simulink model "ffb_Cularis_server"  (Simulink 8.6)
settings: Solver=FixedStepAuto  SolverMode=SingleTasking  StartTime=0.0  StopTime=uavsim.simConfig.tsim  FixedStep=uavsim.simConfig.tsample_model  RelTol=1
model workspace (MAT data in the model file):
  VortexSig = Simulink.Signal
  VortexSig.DataType = 'Bus: VortexStates'
  VortexSig.Units = 'auto'
  VortexSig.Dimensions = [10 1]
  VortexSig.DimensionsMode = 'Fixed'
  VortexSig.Complexity = 'real'
  VortexSig.SampleTime = -1
  VortexSig.SamplingMode = 'auto'
  VortexSig.InitialValue = 'VortexStates_MATLABStruct_array'
undefined symbols (not defined in the file or in its folder): uavsim
libraries: uavsimblockset x4, aerolibtransform2 x4, uavsimBlockset_UAV3DInterface x2, aerolibanimutils x1
settings Model: Creator=mstolle  LastModifiedBy=j.bolting  ExtModeTrigDuration=100
settings SolverCC: ZcThreshold=1e-5  ZeroCrossAlgorithm=Adaptive  AlgebraicLoopSolver=LineSearch  AutoInsertRateTranBlk=on
settings DataIOCC: LimitDataPoints=off  SaveFinalState=on  SaveFormat=StructureWithTime  SignalLoggingSaveFormat=Dataset  SaveOutput=off  SaveState=on  DSMLogging=off  InspectSignalLogs=on  StateSaveName=tmp_raccel_xout
settings OptimizationCC: BlockReduction=off  OptimizeBlockIOStorage=off  BufferReuse=off  GlobalBufferReuse=off  ExpressionFolding=off  LocalBlockOutputs=off  EfficientMapNaN2IntZero=off  SimCompilerOptimization=on
settings DebuggingCC: UnderspecifiedInitializationDetection=Simplified  MergeDetectMultiDrivingBlocksExec=error  IgnoredZcDiagnostic=none  FcnCallInpInsideContextMsg=EnableAllAsError  BusObjectLabelMismatch=error
settings HardwareCC: TargetBitPerPointer=64  TargetLongLongMode=on  TargetIntDivRoundTo=Zero  TargetEndianess=LittleEndian  TargetWordSize=64  TargetHWDeviceType=MATLAB Host  ProdEqTarget=off
settings ModelReferenceCC: UpdateModelReferenceTargets=IfOutOfDate  ModelReferenceNumInstancesAllowed=Single  ModelReferenceMinAlgLoopOccurrences=on
settings SFSimCC: SFSimEcho=off
settings RTWCC: SystemTargetFile=raccel.tlc  TemplateMakefile=raccel_default_tmf  RTWVerbose=off  RTWUseSimCustomCode=on
settings CodeAppCC: GenerateComments=off  MaxIdLength=128  SimulinkBlockComments=off
settings RaccelTargetCC: ERTMultiwordTypeDef=System defined  ERTMultiwordLength=256  GeneratePreprocessorConditionals=Use local settings  ERTFirstTimeCompliant=off  MultiInstanceERTCode=off  ENABLE_SLEXEC_SSBRIDGE=0  RTWCAPIParams=on
settings ConfigComp: CovSFcnEnable=off
settings ConfigurationSet: Description=SimMechanics 2G

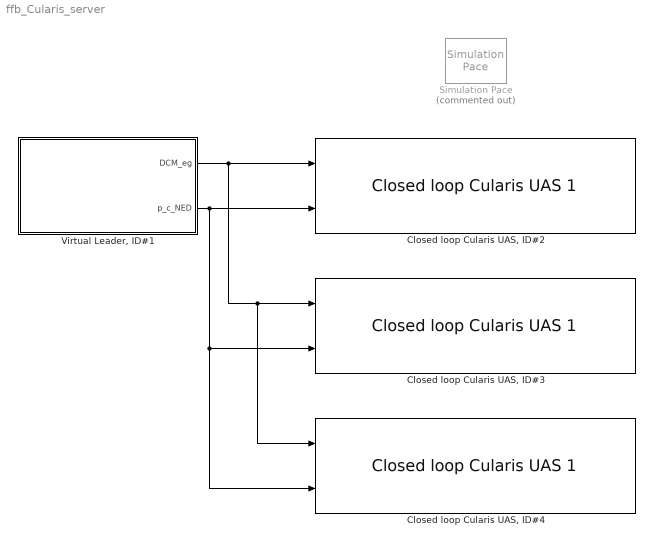
== system ffb_Cularis_server ==
  "Closed loop Cularis UAS, ID#2" : uavsimblockset/Closed loop Cularis UAS 1  closedloopmask_ID=2
  "Closed loop Cularis UAS, ID#3" : uavsimblockset/Closed loop Cularis UAS 1  closedloopmask_ID=3
  "Closed loop Cularis UAS, ID#4" : uavsimblockset/Closed loop Cularis UAS 1  closedloopmask_ID=4
  Simulation Pace : aerolibanimutils/Simulation Pace  Commented=on  SimulationPace=1  SleepMode=MATLAB Thread  OutputPaceError=off  SampleTime=-1
  "Virtual Leader, ID#1" : Subsystem  mask{aircraftmask_phithetapsi0=uavsim.formation(1).phithetapsi0, aircraftmask_p0_NED_m=uavsim.formation(1).p0_NED', aircraftmask_originNED_ECEF_rrm=uavsim.originNED_ECEF_radradm, aircraftmask_pqr0=uavsim.formation(1).omega0, aircraftmask_uvw0=uavsim.formation(1).uvw0, aircraftmask_phithetapsi_trim=uavsim.formation(1).phithetapsi0, aircraftmask_ID=1, aircraftmask_wakevortexenabled=on, aircraftmask_navigationLaw=-1, uavsim=uavsim, leaderID=0, airkraftmask_displayLeader=on}
      mask prompts: aircraftmask_phithetapsi0 "Initial Euler angles [rad]"; aircraftmask_p0_NED_m "Initial position, NED frame [m]"; aircraftmask_originNED_ECEF_rrm "Origin NED frame. ECEF, [rad rad m]"; aircraftmask_pqr0 "Initial rotation rates, body frame [rad/s]"; aircraftmask_uvw0 "Initial velocity, body frame [m/s]"; aircraftmask_phithetapsi_trim "Trim Euler angles [rad]"; aircraftmask_ID "Aircraft ID"; aircraftmask_wakevortexenabled "Wake vortex interaction enabled"; aircraftmask_navigationLaw "Active navigation law (-1: automatic selection)"; uavsim "Parameter set"; leaderID "Follows which ID?"; airkraftmask_displayLeader "Display virtual leader"
      mask Display:
      | % Set Icon:
      | %image(imread('images/cularis.png'), [.2, .2, .6, .6])
  wires:
  "Virtual Leader, ID#1"/1(DCM_eg) -> "Closed loop Cularis UAS, ID#2"/1, "Closed loop Cularis UAS, ID#4"/1, "Closed loop Cularis UAS, ID#3"/1
  "Virtual Leader, ID#1"/2(p_c_NED) -> "Closed loop Cularis UAS, ID#2"/2, "Closed loop Cularis UAS, ID#4"/2, "Closed loop Cularis UAS, ID#3"/2

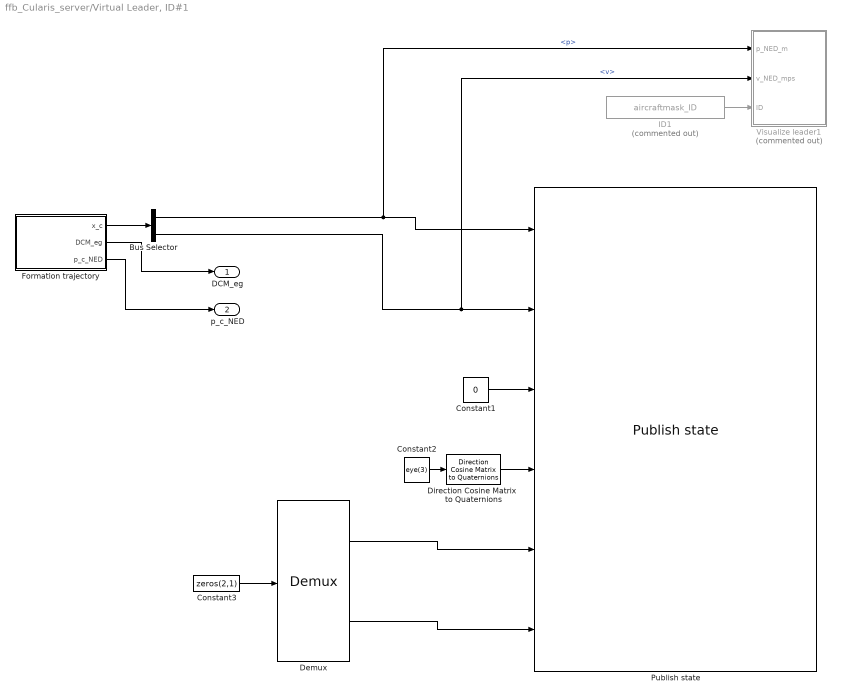
== system ffb_Cularis_server/Virtual Leader, ID#1 ==
  Bus Selector : BusSelector  OutputSignals=p,v
  Constant1 : Constant  Value=0
  Constant2 : Constant  Value=eye(3)
  Constant3 : Constant  Value=zeros(2,1)
  Demux : Demux  Outputs=2
  Direction Cosine Matrix  to Quaternions : aerolibtransform2/Direction Cosine Matrix  to Quaternions
  Formation trajectory : Subsystem
  ID1 : Constant  Commented=on  Value=aircraftmask_ID
  Publish state : uavsimblockset/Publish state  mask_ID=aircraftmask_ID
  Visualize leader1 : Subsystem  Commented=on  AncestorBlock=formationFlyingBlockset/Visualize leader  TreatAsAtomicUnit=on  SystemSampleTime=uavsim.simConfig.tsample_UAV3D  mask{mask_3dmodel=1}
      mask prompts: mask_3dmodel "3D model"
      mask TypeOptions mask_3dmodel: 0 | 1 | 2 | 3
  DCM_eg : Outport
  p_c_NED : Outport  Port=2
  wires:
  Constant1/1 -> Publish state/3
  Bus Selector/1 -> Publish state/1, Visualize leader1/1(p_NED_m)  "<p>"
  Bus Selector/2 -> Publish state/2, Visualize leader1/2(v_NED_mps)  "<v>"
  Direction Cosine Matrix  to Quaternions/1 -> Publish state/4
  Demux/2 -> Publish state/6
  Demux/1 -> Publish state/5
  Constant2/1 -> Direction Cosine Matrix  to Quaternions/1
  Constant3/1 -> Demux/1
  ID1/1 -> Visualize leader1/3(ID)
  Formation trajectory/1(x_c) -> Bus Selector/1
  Formation trajectory/2(DCM_eg) -> DCM_eg/1
  Formation trajectory/3(p_c_NED) -> p_c_NED/1

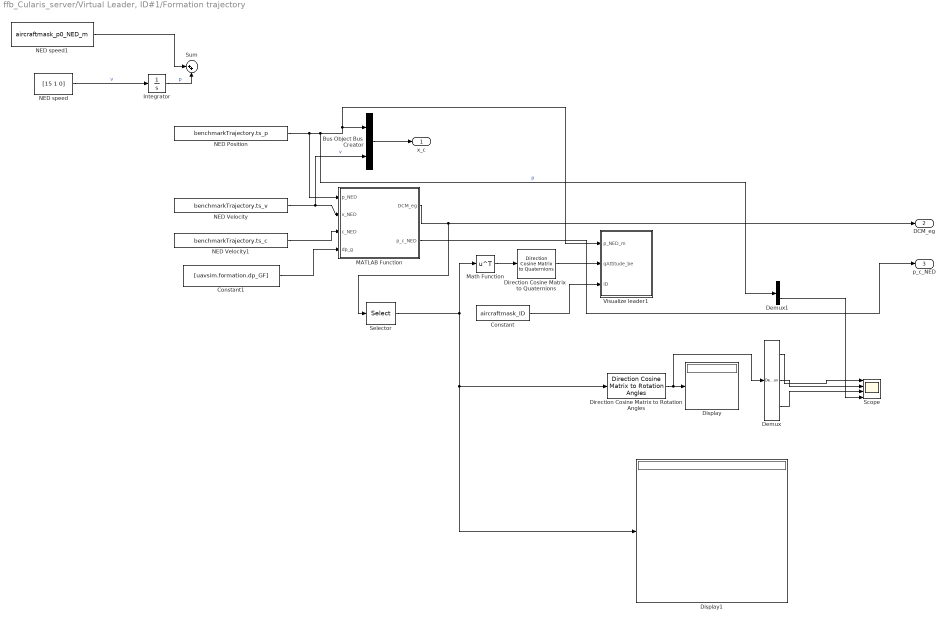
== system ffb_Cularis_server/Virtual Leader, ID#1/Formation trajectory ==
  Bus Object Bus Creator : BusCreator  Inputs=2  OutDataTypeStr=Bus: svm_bus_x  mask(BUS OBJECT Bus Creator){busType=Bus: svm_bus_x}
      mask prompts: busType "Bus Type"
      mask help:
      | Provides users the cabability to painlessly, instantly customize bus creators of output data type 'Bus:' by selecting the bus object type from a drop down menu dynamically populated by bus objects in the workspace.
      |
      | After pressing the "Apply Selection" button signal lines into the creator are populated and named with the elements in the chosen bus saving the user from having to recall and fill out signal line names.
      |
      | NOTE that when copying a Bus Object Bus Creator from your locked Library the link to the Library is automatically broken. This saves the user from having to Unlock Links To Library (From the Library menu.), Disable Link and finally Break Link (Both from the Model menu.) for every placed instance of the block.
      settings: AttributesFormatString=%<OutDataTypeStr>  CopyFcn=set_param(gcb, 'LinkStatus', 'none')
      mask TypeOptions busType: Bus: AHRS | Bus: Acceleration | Bus: Aero | Bus: Airdata | Bus: Airframe | Bus: Attitude | Bus: CMD | Bus: ControlInfoBus | Bus: Dx | Bus: Enginedata | Bus: Environment | Bus: FlightGearData | Bus: GCSUpstream | Bus: GNSSL1 | Bus: GNSSRTK | Bus: GPS | Bus: IMU | Bus: Kinematics | Bus: LandinggearInput | Bus: MotionTracker | Bus: Position | Bus: Radiodistance | Bus: RotationalAcceleration | Bus: RotationalVelocity | Bus: SensorBus | Bus: StateBus | Bus: Velocity | Bus: VortexParameterBus | Bus: VortexStates | Bus: WindAngles | Bus: iUAScom | Bus: svm_bus_d_exo | Bus: svm_bus_u | Bus: svm_bus_x | Bus: svm_bus_xi
      mask Callback busType:
      | % Using variable names terminated with "_BOBC" to lessen the chances of
      | % collisions with existing workspace variables.
      | 
      | % Get the current block handle and mask handle.
      | handleCreator_BOBC = gcbh;
      | maskObj_BOBC       = Simulink.Mask.get(gcb);
      | 
      | % Get a list of variables in the workspace in order to search for the '1x1
      | % Bus' types.
      | wsVars_BOBC = whos;
      | 
      | % Reset the 'TypeOptions' bus list in case some '1x1 Bus' types have been
      | % deleted from or added to the workspace.
      | maskObj_BOBC.Parameters.TypeOptions = {'<empty>'};
      | 
      | % Reset the bus count.
      | busCount_BOBC = 0;
      | 
      | for index_BOBC = 1:length(wsVars_BOBC)
      | 
      |    % If the variable is a bus object...
      |    if strcmp(wsVars_BOBC(index_BOBC).class, 'Simulink.Bus')
      | 
      |       busCount_BOBC = busCount_BOBC + 1;
      | 
      |       % ... add it to the TypeOptions of the mask.
      |       maskObj_BOBC.Parameters.TypeOptions(busCount_BOBC) = ...
      |                                                            ...
      |                                  {['Bus: ', wsVars_BOBC(index_BOBC).name]};
      |    end
      | end
      | 
      | if busCount_BOBC == 0
      | 
      |    % If there are NO bus objects in the workspace then provide a warning
      |    % popup...
      |    warndlg('There are currently no bus objects in the workspace - you have no use for this block. Use a normal Bus Creator instead.')
      | 
      |    % ... and do nothing.
      | elseif ~strcmp(get_param(handleCreator_BOBC, 'OutDataTypeStr'), 'Inherit: auto')
      | 
      |    % If the currently selected bus data type ('OutDataTypeStr') is not
      |    % 'Inherit: auto' (i.e., if we are reopening the mask.) then get the
      |    % current 'OutDataTypeStr' and 'maskVal.' ('maskVal' is the selected
      |    % 'TypeOptions' list member.)
      |    outDatStr_BOBC = get_param(handleCreator_BOBC, 'OutDataTypeStr');
      |    maskVal_BOBC   = get_param(handleCreator_BOBC, 'MaskValues');
      | 
      |    if ~strcmp(outDatStr_BOBC, maskVal_BOBC{1})
      | 
      |       % Upon re-opening the mask if the default 'TypeOptions' list member
      |       % (The first one.) contained in 'maskVal' does not match the
      |       % currently selected bus data type ('OutDataTypeStr') then set the
      |       % 'TypeOptions' list member to the selected bus data type. (Cuts down
      |       % on confusion to have the displayed list member match the selected
      |       % bus data type rather than the first entry.)
      |       set_param(handleCreator_BOBC, 'MaskValues', {outDatStr_BOBC});
      |    end
      | end
      | 
      | % Clean up the workspace.
      | clear  handleCreator_BOBC  maskObj_BOBC     wsVars_BOBC ...
      |             busCount_BOBC    index_BOBC  outDatStr_BOBC ...
      |              maskVal_BOBC
      mask DialogControl applyMOCBSelection Prompt: Apply Selection
      mask DialogControl applyMOCBSelection Callback:
      | % Using variable names terminated with "_BOBC" to lessen the chances of
      | % collisions with existing workspace variables.
      | 
      | % Get the current block, current block handle and mask handle.
      | currentBlock_BOBC  = gcb;
      | handleCreator_BOBC = gcbh;
      | 
      | % Get the desired bus type...
      | desiredBusType_BOBC = get_param(handleCreator_BOBC, 'busType');
      | 
      | % ... and set the 'OutDataTypeStr' to it.
      | set_param(handleCreator_BOBC, 'OutDataTypeStr', desiredBusType_BOBC);
      | 
      | %% First delete any existing lines on the port.
      | % Get the line handles.
      | lh_BOBC = get_param(handleCreator_BOBC, 'LineHandles');
      | 
      | % If any lines exist (Non- -1 line handles.), delete them and start over.
      | if max(lh_BOBC.Inport > 0)
      | 
      |    for index_BOBC = 1:length(lh_BOBC.Inport)
      | 
      |       if lh_BOBC.Inport(index_BOBC) > 0
      | 
      |          delete_line(lh_BOBC.Inport(index_BOBC))
      |       end
      |    end
      | end
      | 
      | %% Then work on adding new lines.
      | 
      | % Get the block path for 'add_line' function.
      | blockPath_BOBC = get_param(handleCreator_BOBC, 'Parent');
      | 
      | % Get the newly selected bus type ('OutDataTypeStr')...
      | mocbBusType_BOBC = get_param(currentBlock_BOBC, 'OutDataTypeStr');
      | 
      | % ... and parse off "Bus: " so the string of the desired bus contained in
      | % 'OutDataTypeStr' matches the raw workspace bus names.
      | mocbBusType_BOBC = mocbBusType_BOBC(6:end);
      | 
      | % Then evaluate the string containing the workspace bus name which will
      | % load the desired bus parameters.
      | busParams_BOBC = eval(mocbBusType_BOBC);
      | 
      | % From the parameters grab the number of lines to add.
      | numLines_BOBC = length(busParams_BOBC.Elements);
      | 
      | % Set the number of inputs of the masked bus creator to the number of lines
      | % to add.
      | set_param(handleCreator_BOBC, 'Inputs', num2str(numLines_BOBC));
      | 
      | % Get (Inputs.) port handles so we can grab the positions of them.
      | ph_BOBC = get_param(handleCreator_BOBC, 'PortHandles');
      | 
      | for index_BOBC = 1:numLines_BOBC
      | 
      |    % Get the position of input port number 'index_BOBC'.
      |    portPos_BOBC = get_param(ph_BOBC.Inport(index_BOBC), 'Position');
      | 
      |    % Add a line from 50 pixels left of the port position to the port
      |    % position. (This must be done because it's the lines that get named,
      |    % not the port positions.)
      |    portLine_BOBC = add_line(blockPath_BOBC, [portPos_BOBC - [50 0]; portPos_BOBC]);
      | 
      |    % Rename the new line to the bus 'index_BOBC-st/nd/rd/th' element name.
      |    set_param(portLine_BOBC, 'Name', busParams_BOBC.Elements(index_BOBC).Name)
      | end
      | 
      | %% Cleanup the workspace.
      | clear    currentBlock_BOBC  handleCreator_BOBC      index_BOBC ...
      |        desiredBusType_BOBC             lh_BOBC  blockPath_BOBC ...
      |           mocbBusType_BOBC      busParams_BOBC   numLines_BOBC ...
      |                    ph_BOBC        portPos_BOBC   portLine_BOBC
  Constant : Constant  Value=aircraftmask_ID
  Constant1 : Constant  Value=[uavsim.formation.dp_GF]
  Demux : Demux  Outputs=3
  Demux1 : Demux  Outputs=3
  Direction Cosine Matrix to Rotation Angles : aerolibtransform2/Direction Cosine Matrix to Rotation Angles  rotationOrder=ZYX  lim=Default
      settings: AttributesFormatString=Rotation Order: %<rotationOrder>
  Direction Cosine Matrix  to Quaternions : aerolibtransform2/Direction Cosine Matrix  to Quaternions
  Display : Display
      settings: Decimation=3
  Display1 : Display
      settings: Decimation=3
  Integrator : Integrator  InitialCondition=[0 0 0]
  MATLAB Function : MATLAB Function  TreatAsAtomicUnit=on
  Math Function : Math  Operator=transpose  SaturateOnIntegerOverflow=on
  NED Position : FromWorkspace  VariableName=benchmarkTrajectory.ts_p  SampleTime=0
  NED Velocity : FromWorkspace  VariableName=benchmarkTrajectory.ts_v  SampleTime=0
  NED Velocity1 : FromWorkspace  VariableName=benchmarkTrajectory.ts_c  SampleTime=0
  NED speed : Constant  Value=[15 1 0]
  NED speed1 : Constant  Value=aircraftmask_p0_NED_m
  Scope : Scope  NumInputPorts=4
  Selector : Selector  NumberOfDimensions=3  InputPortWidth=3  IndexOptions=Index vector (dialog),Index vector (dialog),Index vector (dialog)  Indices=1:3,1:3,1  OutputSizes=1,1,1
  Sum : Sum  Inputs=|++
  Visualize leader1 : Subsystem  TreatAsAtomicUnit=on  SystemSampleTime=uavsim.simConfig.tsample_UAV3D  mask{mask_3dmodel=3}
      mask prompts: mask_3dmodel "3D model"
      mask TypeOptions mask_3dmodel: 0 | 1 | 2 | 3
  x_c : Outport  OutDataTypeStr=Bus: svm_bus_x
  DCM_eg : Outport  Port=2
  p_c_NED : Outport  Port=3
  wires:
  NED Position/1 -> MATLAB Function/1(p_NED), Demux1/1, Visualize leader1/1(p_NED_m), Bus Object Bus Creator/1  "p"
  NED speed/1 -> Integrator/1  "v"
  Bus Object Bus Creator/1 -> x_c/1
  Integrator/1 -> Sum/2  "p"
  NED speed1/1 -> Sum/1
  NED Velocity/1 -> MATLAB Function/2(v_NED), Bus Object Bus Creator/2  "v"
  NED Velocity1/1 -> MATLAB Function/3(c_NED)
  Selector/1 -> Display1/1, Direction Cosine Matrix to Rotation Angles/1, Math Function/1
  Direction Cosine Matrix  to Quaternions/1 -> Visualize leader1/2(qAttitude_be)
  Constant/1 -> Visualize leader1/3(ID)
  Direction Cosine Matrix to Rotation Angles/1 -> Demux/1, Display/1
  Demux/2 -> Scope/2
  Demux/3 -> Scope/3
  Demux/1 -> Scope/1
  Demux1/3 -> Scope/4
  Constant1/1 -> MATLAB Function/4(dp_g)
  MATLAB Function/1(DCM_eg) -> Selector/1, DCM_eg/1
  MATLAB Function/2(p_c_NED) -> p_c_NED/1
  Math Function/1 -> Direction Cosine Matrix  to Quaternions/1

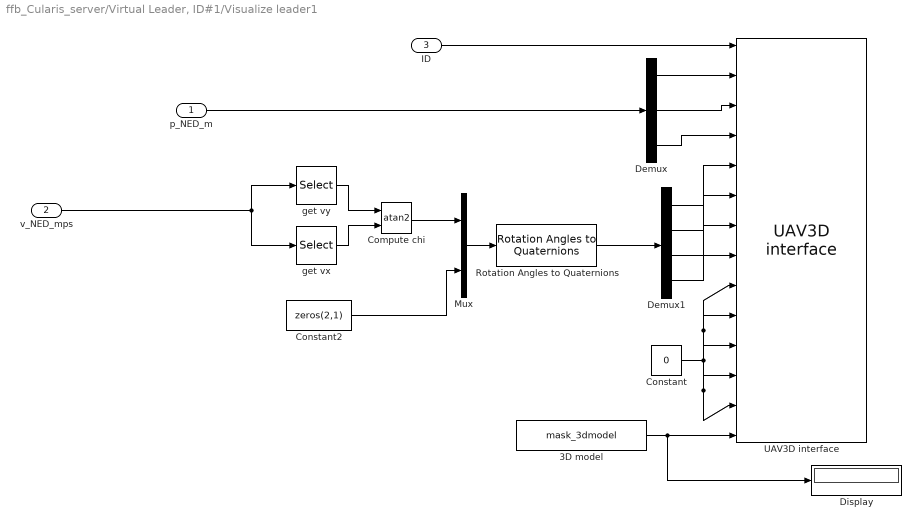
== system ffb_Cularis_server/Virtual Leader, ID#1/Visualize leader1 ==
  p_NED_m : Inport
  v_NED_mps : Inport  Port=2
  ID : Inport  Port=3
  3D model : Constant  Value=mask_3dmodel
  Compute chi : Trigonometry  Operator=atan2
  Constant : Constant  Value=0
  Constant2 : Constant  Value=zeros(2,1)
  Demux : Demux  Outputs=3
  Demux1 : Demux
  Display : Display
  Mux : Mux  Inputs=2
  Rotation Angles to Quaternions : aerolibtransform2/Rotation Angles to Quaternions  rotationOrder=ZYX
  UAV3D interface : uavsimBlockset_UAV3DInterface/UAV3D interface  ip='localhost'  udpport=4445
  get vx : Selector  InputPortWidth=3  IndexOptions=Index vector (dialog)  Indices=1  OutputSizes=1
  get vy : Selector  InputPortWidth=3  IndexOptions=Index vector (dialog)  Indices=2  OutputSizes=1
  wires:
  Demux/1 -> UAV3D interface/2
  Demux/2 -> UAV3D interface/3
  Demux/3 -> UAV3D interface/4
  Demux1/1 -> UAV3D interface/5
  Demux1/2 -> UAV3D interface/6
  Demux1/4 -> UAV3D interface/8
  get vy/1 -> Compute chi/1
  get vx/1 -> Compute chi/2
  Constant2/1 -> Mux/2
  Mux/1 -> Rotation Angles to Quaternions/1
  Rotation Angles to Quaternions/1 -> Demux1/1
  Compute chi/1 -> Mux/1
  Demux1/3 -> UAV3D interface/7
  Constant/1 -> UAV3D interface/13, UAV3D interface/12, UAV3D interface/11, UAV3D interface/10, UAV3D interface/9
  3D model/1 -> Display/1, UAV3D interface/14
  ID/1 -> UAV3D interface/1
  p_NED_m/1 -> Demux/1
  v_NED_mps/1 -> get vy/1, get vx/1

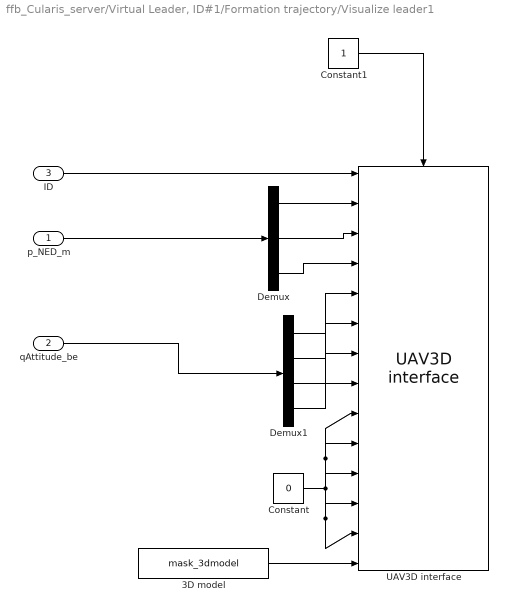
== system ffb_Cularis_server/Virtual Leader, ID#1/Formation trajectory/Visualize leader1 ==
  p_NED_m : Inport
  qAttitude_be : Inport  Port=2
  ID : Inport  Port=3
  3D model : Constant  Value=mask_3dmodel
  Constant : Constant  Value=0
  Constant1 : Constant
  Demux : Demux  Outputs=3
  Demux1 : Demux
  UAV3D interface : uavsimBlockset_UAV3DInterface/UAV3D interface  ip='localhost'  udpport=4445
  wires:
  Demux/1 -> UAV3D interface/2
  Demux/2 -> UAV3D interface/3
  Demux/3 -> UAV3D interface/4
  Demux1/1 -> UAV3D interface/5
  Demux1/2 -> UAV3D interface/6
  Demux1/4 -> UAV3D interface/8
  qAttitude_be/1 -> Demux1/1
  Demux1/3 -> UAV3D interface/7
  Constant/1 -> UAV3D interface/13, UAV3D interface/12, UAV3D interface/11, UAV3D interface/10, UAV3D interface/9
  3D model/1 -> UAV3D interface/14
  ID/1 -> UAV3D interface/1
  p_NED_m/1 -> Demux/1
  Constant1/1 -> UAV3D interface/Enable

== matlab function Virtual Leader, ID#1/Formation trajectory/MATLAB Function ==
  data: p_NED input double; v_NED input double; DCM_eg output double; c_NED input double; dp_g input double; p_c_NED output double
% Compute the DCM between the formation guidance frame (g) and the NED
% frame (e) for each UAS from the trajectory velocity and curvature vectors
% and the separation vectors between UAS.
function [DCM_eg, p_c_NED] = computeDCM_eg(p_NED,v_NED, c_NED, dp_g)
%#codegen
persistent last_uz;
if isempty(last_uz)
    last_uz = repmat([0 0 -1]', 1, 10);
end
p_c_NED = zeros(3,10);

% Compute the centripetal acceleration of the virtual leader:
% radius of the leader's instantaneous orbit:
a_centrip = zeros(3,1);
omega_vl = [0 0 0]';
if norm(c_NED) > eps
    r_vl = 1/(norm(c_NED));
    ur = -fflib_normalize(c_NED);
    omega_vl = cross(r_vl*ur, v_NED)/(r_vl^2);
    a_centrip = norm(omega_vl)^2 * r_vl*ur;
    bp = 0;
end

ux = fflib_normalize(v_NED);
[uz, last_uz] = compute_uz(ux, a_centrip, last_uz);

uy = cross(uz, ux);
DCM_eg = zeros(3,3,10);
DCM_eg(:, :, 1) = [ux uy uz];

% compute DCMs for remaining UASs's:
pddot_pre = a_centrip;
pdot_pre = v_NED;
omega_pre = omega_vl;
p_c_NED(:, 1) = p_NED;
for k=1:size(dp_g, 2)-1
    dp_e = DCM_eg(:, :, k) * dp_g(:, k);
    p_c_NED(:, k+1) = p_c_NED(:, k) + dp_e;
    pdot_fol = pdot_pre + cross(omega_pre, dp_e);
    pddot_fol = pddot_pre + cross(omega_pre, cross(omega_pre, dp_e));
    omega_fol_norm = (norm(pddot_fol)/norm(dp_e))^(1/2);
    omega_fol = omega_fol_norm * fflib_normalize(cross(pddot_fol, pdot_fol));
    if ~isempty(find(isnan(norm(omega_fol)), 1))
        omega_fol = zeros(3,1);
    end
    ux = fflib_normalize(pdot_fol);
    [uz, last_uz] = compute_uz(ux, pddot_fol, last_uz);
    uy = cross(uz, ux);
    DCM_eg(:, :, k+1) = [ux uy uz];
    pddot_pre = pddot_fol;
    pdot_pre = pdot_fol;
    omega_pre = omega_fol;
    bp = 0;
end
bp = 0;
end

function [uz, last_uz] = compute_uz(ux, a_centrip, lastuz_in)
last_uz = lastuz_in;
a_total = [0 0 9.81]' + a_centrip;
% Compute acceleration vector projected on y-z plane of the g frame:
a_total_yz = ffb_projectVectorOnPlane(a_total, ux);
% Total force defines z axis:
if norm(a_total_yz) > eps
    uz = fflib_normalize(a_total_yz);
    last_uz(:, 1) = uz;
else
    uz = lastuz_in(:, 1);
end
if uz(3) < 0
    bp = 0;
    uz = -uz;
end

end
